simulink model "cc_cv"  (R2024a)
settings: Solver=VariableStepAuto  StartTime=0.0  StopTime=10  RelTol=1e-3
undefined symbols (not defined in the file): Ion, Lithium
libraries: spsBreakerLib x2, spsBatteryLib x1, spsControlledCurrentSourceLib x1, spsDCVoltageSourceLib x1, simulink x1, spsSeriesRLCBranchLib x1, sps_lib x1
settings Model: Creator=gades  LastModifiedBy=gades

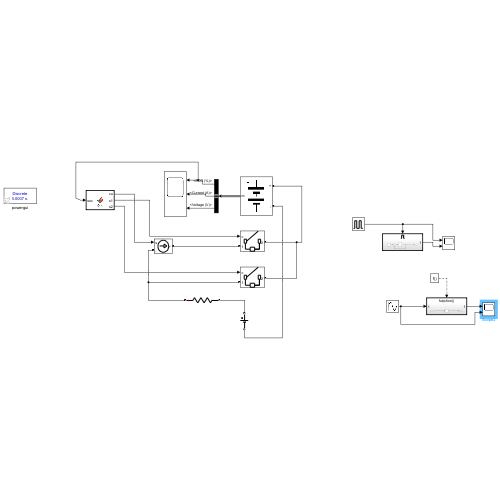
[thumbnail: Simulink's stored preview of the top-level diagram]
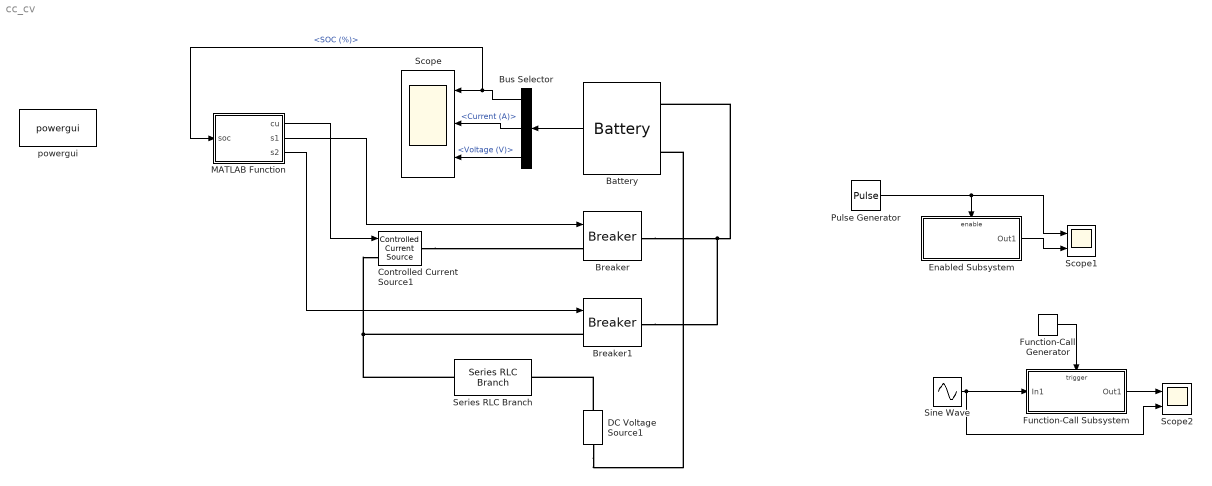
== system cc_cv ==
  Battery : spsBatteryLib/Battery  BatType=Lithium-Ion  ShowTempParam=off  ThermalPreset=no  ShowAgeParam=off  NomV=12  NomQ=6  SOC=65  Batt_Tr=30  PresetModel=on  MaxQ=6  MinV=9  FullV=13.9678  Dis_rate=2.6087  R=0.02  Normal_OP=5.4261  expZone="[12.9646     0.294783]"  current=[6.5 13 32.5]  Units=Time  Tci=20  NomT=20  T2=-30  MaxQ2=4.8  FullV2=7.1  Normal_OP2=5.655  expZone2="[6.58           1]"  Rca=0.6  ti=2000  Dp=0  Neq0=0  Tsim=1e6  Ta1=25  Qeol=5.4*0.9  Reol=0.013333*1.2  Char_age=[2.3478, 3]  Dis_age=[2.3478, 10]  N1=1500  N2=10500  N3=1000  N4=1400  Ta2=45  N5=950
  Breaker : spsBreakerLib/Breaker  InitialState=0  SwitchingTimes="[1/60  5/60]"  External=on  BreakerResistance=0.01  SnubberResistance=1e6  SnubberCapacitance=inf  Measurements=None  MoreParameters=on  NoBreakLoop=off
  Breaker1 : spsBreakerLib/Breaker  InitialState=0  SwitchingTimes="[1/60  5/60]"  External=on  BreakerResistance=0.01  SnubberResistance=1e6  SnubberCapacitance=inf  Measurements=None  MoreParameters=on  NoBreakLoop=off
  Bus Selector : BusSelector  OutputSignals=SOC (%),Current (A),Voltage (V)
  Controlled Current Source1 : spsControlledCurrentSourceLib/Controlled Current Source  Initialize=on  Source_Type=AC  Amplitude=0  Phase=0  Frequency=0  Measurements=None
  DC Voltage Source1 : spsDCVoltageSourceLib/DC Voltage Source  Amplitude=13.5  Measurements=None
  Enabled Subsystem : Subsystem  TreatAsAtomicUnit=on
  Function-Call Generator : simulink/Ports & Subsystems/Function-Call Generator  sample_time=0.01  numberOfIterations=1  DisallowWideOutput=off
  Function-Call Subsystem : Subsystem  TreatAsAtomicUnit=on
  MATLAB Function : MATLAB Function  TreatAsAtomicUnit=on
  Pulse Generator : DiscretePulseGenerator  PulseType=Time based  Period=4  PulseWidth=50  PhaseDelay=1
  Scope : Scope  NumInputPorts=3
  Scope1 : Scope  NumInputPorts=2
  Scope2 : Scope  NumInputPorts=2
  Series RLC Branch : spsSeriesRLCBranchLib/Series RLC Branch  LConnTagsString=__new0  RConnTagsString=__new0  BranchType=R  Resistance=0.001  Inductance=1e-3  SetiL0=off  InitialCurrent=0  Capacitance=1e-6  Setx0=off  InitialVoltage=0  Measurements=None
  Sine Wave : Sin  SampleTime=0
  powergui : sps_lib/powergui  Priority=1  SimulationMode=Discrete  SampleTime=700e-6  frequency=60  Iterations=50  frequencyindice=0  Pbase=100e6  ErrMax=1e-4  UnitsV=kV  UnitsW=MW  buscounter=0  FunctionMessages=off  echomessages=off  EnableUseOfTLC=off  CurrentSourceSwitches=off  DisableSnubberDevices=off  DisableRonSwitches=off  DisableVfSwitches=off  DisplayEquations=off  AutomaticDiscreteSolvers=off  SolverType=Tustin/Backward Euler (TBE)  Interpol=off  ExternalGateDelay=off  methode=off  Ts=100  x0status=blocks  SPID=on  SwTol=0  HookPort=off  NonlinearTolerance=1e-4  nMaxIteration=100  ContinueOnMaxIteration=off  RestoreLinks=warning  ResistiveCurrentMeasurement=off  Frange=[0:2:500]  Ylog=off  Xlog=on  ShowGrid=off  save=off  variable=ZData  structure=0  ZoomFFT=off  StartTime=0.0  cycles=1  DisplayStyle=1  fundamental=60  FreqAxis=off  MaxFrequency=1000  frequencyindicesteady=1  RmsSteady=1  display=off
  wires:
  Battery/1 -> Bus Selector/1
  Bus Selector/2 -> Scope/2  "<Current (A)>"
  Bus Selector/1 -> MATLAB Function/1(soc), Scope/1  "<SOC (%)>"
  Bus Selector/3 -> Scope/3  "<Voltage (V)>"
  MATLAB Function/1(cu) -> Controlled Current Source1/1
  MATLAB Function/2(s1) -> Breaker/1
  MATLAB Function/3(s2) -> Breaker1/1
  Pulse Generator/1 -> Scope1/1, Enabled Subsystem/Enable
  Enabled Subsystem/1(Out1) -> Scope1/2
  Function-Call Generator/1 -> Function-Call Subsystem/Trigger
  Function-Call Subsystem/1(Out1) -> Scope2/1
  Sine Wave/1 -> Scope2/2, Function-Call Subsystem/1(In1)
  connections:
  DC Voltage Source1/RConn1 -- Series RLC Branch/RConn1
  Breaker/RConn1 -- Breaker1/RConn1 -- Battery/LConn1
  DC Voltage Source1/LConn1 -- Battery/LConn2
  Controlled Current Source1/RConn1 -- Breaker/LConn1
  Series RLC Branch/LConn1 -- Breaker1/LConn1 -- Controlled Current Source1/LConn1

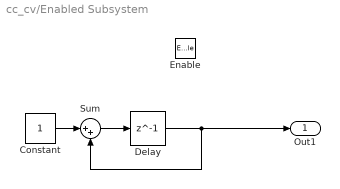
== system cc_cv/Enabled Subsystem ==
  Enable : EnablePort  StatesWhenEnabling=reset
  Constant : Constant
  Delay : Delay  DelayLength=1
  Sum : Sum  Inputs=|++
  Out1 : Outport
  wires:
  Constant/1 -> Sum/1
  Sum/1 -> Delay/1
  Delay/1 -> Sum/2, Out1/1

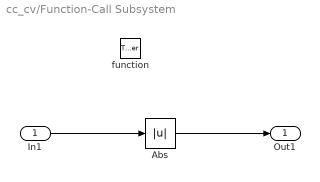
== system cc_cv/Function-Call Subsystem ==
  In1 : Inport
  function : TriggerPort  TriggerType=function-call  VariantControl=(inherit)
  Abs : Abs  SaturateOnIntegerOverflow=off
  Out1 : Outport
  wires:
  In1/1 -> Abs/1
  Abs/1 -> Out1/1

== matlab function cc_cv/MATLAB Function ==
  data: soc input; cu output; s1 output; s2 output
function [cu,s1,s2] = fcn(soc)

 
cu=0
if soc==70||soc<=70
    cu=2;
    s1=1;
    s2=0;
else
    s1=0;
    s2=1;
end


if soc==100
    cu=0;
    s1=0;
    s2=0;
end
